simulink model "serial_arduino"  (R2018b)
settings: Solver=VariableStepAuto  StartTime=0.0  StopTime=inf  RelTol=1e-3
settings Model: Creator=Roberto  LastModifiedBy=Roberto

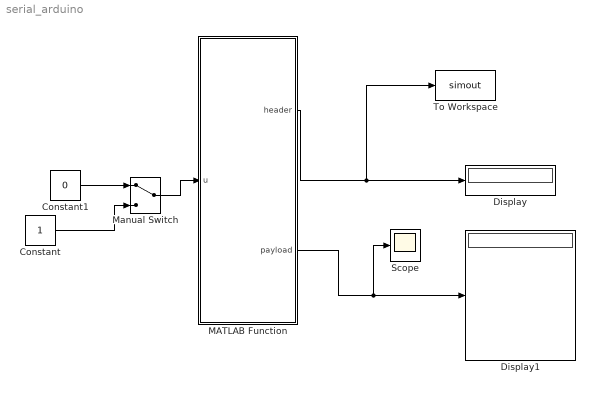
== system serial_arduino ==
  Constant : Constant
  Constant1 : Constant  Value=0
  Display : Display
  Display1 : Display
  MATLAB Function : MATLAB Function  TreatAsAtomicUnit=on
  Manual Switch : ManualSwitch
  Scope : Scope
  To Workspace : ToWorkspace  VariableName=simout  SampleTime=-1
  wires:
  MATLAB Function/1(header) -> Display/1, To Workspace/1
  Manual Switch/1 -> MATLAB Function/1(u)
  Constant1/1 -> Manual Switch/1
  Constant/1 -> Manual Switch/2
  MATLAB Function/2(payload) -> Scope/1, Display1/1

== matlab function serial_arduino/MATLAB Function ==
  data: header output; u input; payload output
function [header ,payload ] = fcn(u)
% [ch1,ch2,ch3,ch4,ch5,ch6,ch7,ch8] = fcn(u)

    a=true;
    header = zeros(2,1);
    payload = zeros(5,1);
    coder.extrinsic('serial', 'fopen','fprintf','get','instrfind','display');
    
    persistent s
    
    
    if isempty(s)

        a=isempty(instrfind);
        if a==0
            fclose(instrfind);
        end

        s = serial('COM4');

        set(s,'InputBufferSize',10000);
        set(s,'BaudRate',115200);
        fopen(s);

        %fprintf(s,'=');

    end

    if u == 0
         header = fread(s,2,'uint8');
         if header(1)==34 && header(2)==66
             payload = fread(s,5,'uint16');
         end
    end
    
     if u > 0
         fclose(s);
     end

end
